simulink model "LIM_version_25052023"  (R2021a)
settings: Solver=VariableStepAuto  StartTime=0.0  StopTime=10.0  RelTol=1e-3
values from neighbouring files (symbols this model uses):
  ki_force = 1    [LIMvariables.m]
  ki_iedx = 80000    [LIMvariables.m]
  ki_ieqx = 80000    [LIMvariables.m]
  ki_lambda = 1000000    [LIMvariables.m]
  ki_speed = 10    [LIMvariables.m]
  kp_force = 0.15    [LIMvariables.m]
  kp_iedx = 25    [LIMvariables.m]
  kp_ieqx = 25    [LIMvariables.m]
  kp_lambda = 200    [LIMvariables.m]
  kp_speed = 0.1    [LIMvariables.m]
  l = 0.308    [LIMvariables.m]
  Llx = 0.0225    [LIMvariables.m]
  Lly = 0.0065    [LIMvariables.m]
  Lm = 0.0416    [LIM_parameters.m]    (also in LIMvariables.m = 0.0376)
  P = 4400    [LIMvariables.m]
  Rx = 1.2    [LIMvariables.m]
  Ry = 2.7    [LIMvariables.m]
  tau = L/p    (= 0.25)    [LIM_parameters.m]    (also in LIMvariables.m = 0.066)
undefined symbols (not defined in the file or in its folder): M, omega_e
libraries: slpidlib x5, simulink x3, simulink_extras x1
settings Model: Creator=Asus  LastModifiedBy=Asus

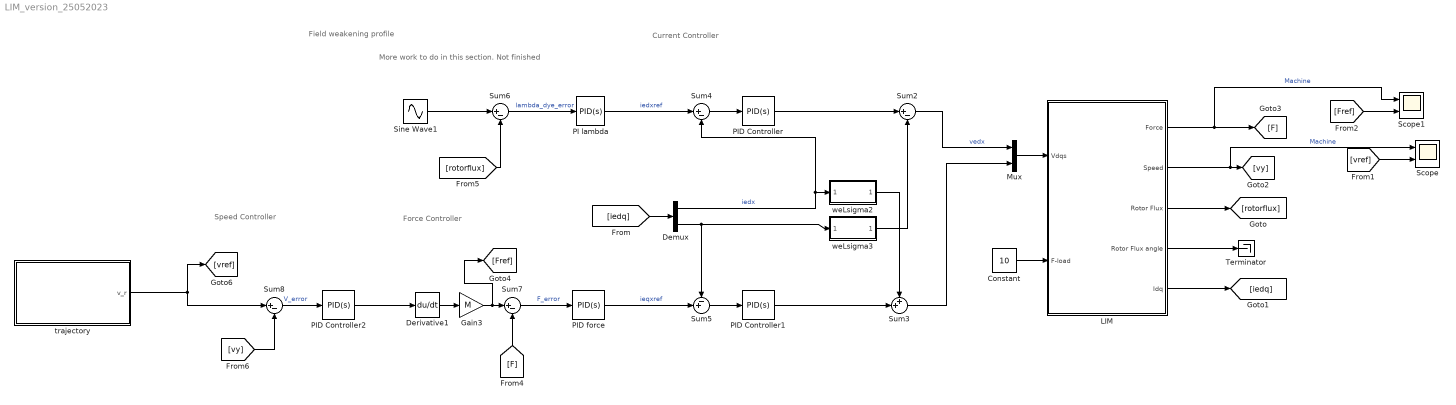
== system LIM_version_25052023 ==
  note: Current Controller
  note: Force Controller
  note: Field weakening profile
  note: Speed Controller
  note: More work to do in this section. Not finished
  Constant : Constant  Value=10
  Demux : Demux  Outputs=2
  Derivative1 : Derivative
  Gain3 : Gain  Gain=M
  LIM : Subsystem
  Mux : Mux  Inputs=2
  PI lambda : slpidlib/PID Controller  Controller=PID  Form=Parallel  TimeDomain=Continuous-time  UseExternalTs=off  SampleTime=-1  IntegratorMethod=Forward Euler  FilterMethod=Forward Euler  ControllerParametersSource=internal  P=kp_lambda  I=ki_lambda  D=0  UseFilter=on  N=100  TunerSelectOption=Transfer Function Based (PID Tuner App)  InitialConditionSource=internal  InitialConditionForIntegrator=0  InitialConditionForFilter=0  DifferentiatorICPrevScaledInput=0  ExternalReset=none  TrackingMode=off  Kt=1  LimitOutput=off  SatLimitsSource=internal  UpperSaturationLimit=inf  LowerSaturationLimit=-inf  LinearizeAsGain=on  AntiWindupMode=none  Kb=1  POutMin=[]  POutMax=[]  IOutMin=[]  IOutMax=[]  DOutMin=[]  DOutMax=[]  NOutMin=[]  NOutMax=[]  SumOutMin=[]  SumOutMax=[]  SaturationOutMin=[]  SaturationOutMax=[]  PParamMin=[]  PParamMax=[]  IParamMin=[]  IParamMax=[]  DParamMin=[]  DParamMax=[]  NParamMin=[]  NParamMax=[]  KbParamMin=[]  KbParamMax=[]  KtParamMin=[]  KtParamMax=[]  KbOutMin=[]  KbOutMax=[]  KtOutMin=[]  KtOutMax=[]  IntegratorOutMin=[]  IntegratorOutMax=[]  FilterOutMin=[]  FilterOutMax=[]  SumI1OutMin=[]  SumI1OutMax=[]  SumI2OutMin=[]  SumI2OutMax=[]  SumI3OutMin=[]  SumI3OutMax=[]  SumI4OutMin=[]  SumI4OutMax=[]  SumDOutMin=[]  SumDOutMax=[]  DifferentiatorOutMin=[]  DifferentiatorOutMax=[]  FilterDiffOutCoefMin=[]  FilterDiffOutCoefMax=[]  ReciprocalOutMin=[]  ReciprocalOutMax=[]  SumDenOutMin=[]  SumDenOutMax=[]  SumNumOutMin=[]  SumNumOutMax=[]  DivideOutMin=[]  DivideOutMax=[]  UdiffTsProdOutMin=[]  UdiffTsProdOutMax=[]  NTsProdOutMin=[]  NTsProdOutMax=[]  UintegralTsProdOutMin=[]  UintegralTsProdOutMax=[]  UngainTsProdOutMin=[]  UngainTsProdOutMax=[]  IntegratorContinuousStateAttributes=''  IntegratorStateMustResolveToSignalObject=off  IntegratorRTWStateStorageClass=Auto  FilterContinuousStateAttributes=''  FilterStateMustResolveToSignalObject=off  FilterRTWStateStorageClass=Auto  ParallelPVariant=InternalParameters  IdealPVariant=Disabled  IVariant=InternalParameters  DVariant=InternalParameters  IntegratorVariant=Continuous  SatVariant=Disabled  AWVariant=Passthrough  PCopyVariant=Disabled  TRVariant=Disabled  FdbkBlocksVariant=Forward  IdealPFdbkVariant=Disabled  SatFdbkVariant=Disabled  DerivativeFilterVariant=ContFilter  NVariant=InternalParameters  NCopyVariant=Disabled  FilterICVariant=InternalICsFilter  IntegratorICVariant=InternalICs  ExternalResetVariant=Disabled  TRSumVariant=Passthrough  SumFdbkVariant=Disabled  SumVariant=Sum_PID  TsampFilterVariant=InternalTs  TsampNgainVariant=Passthrough  TsampIntegralVariant=Passthrough  ExternalSaturationOutDataTypeStr=Inherit: Same as second input
  PID Controller : slpidlib/PID Controller  Controller=PID  Form=Parallel  TimeDomain=Continuous-time  UseExternalTs=off  SampleTime=-1  IntegratorMethod=Forward Euler  FilterMethod=Forward Euler  ControllerParametersSource=internal  P=kp_ieqx  I=ki_ieqx  D=0  UseFilter=on  N=100  TunerSelectOption=Transfer Function Based (PID Tuner App)  InitialConditionSource=internal  InitialConditionForIntegrator=0  InitialConditionForFilter=0  DifferentiatorICPrevScaledInput=0  ExternalReset=none  TrackingMode=off  Kt=1  LimitOutput=off  SatLimitsSource=internal  UpperSaturationLimit=inf  LowerSaturationLimit=-inf  LinearizeAsGain=on  AntiWindupMode=none  Kb=1  POutMin=[]  POutMax=[]  IOutMin=[]  IOutMax=[]  DOutMin=[]  DOutMax=[]  NOutMin=[]  NOutMax=[]  SumOutMin=[]  SumOutMax=[]  SaturationOutMin=[]  SaturationOutMax=[]  PParamMin=[]  PParamMax=[]  IParamMin=[]  IParamMax=[]  DParamMin=[]  DParamMax=[]  NParamMin=[]  NParamMax=[]  KbParamMin=[]  KbParamMax=[]  KtParamMin=[]  KtParamMax=[]  KbOutMin=[]  KbOutMax=[]  KtOutMin=[]  KtOutMax=[]  IntegratorOutMin=[]  IntegratorOutMax=[]  FilterOutMin=[]  FilterOutMax=[]  SumI1OutMin=[]  SumI1OutMax=[]  SumI2OutMin=[]  SumI2OutMax=[]  SumI3OutMin=[]  SumI3OutMax=[]  SumI4OutMin=[]  SumI4OutMax=[]  SumDOutMin=[]  SumDOutMax=[]  DifferentiatorOutMin=[]  DifferentiatorOutMax=[]  FilterDiffOutCoefMin=[]  FilterDiffOutCoefMax=[]  ReciprocalOutMin=[]  ReciprocalOutMax=[]  SumDenOutMin=[]  SumDenOutMax=[]  SumNumOutMin=[]  SumNumOutMax=[]  DivideOutMin=[]  DivideOutMax=[]  UdiffTsProdOutMin=[]  UdiffTsProdOutMax=[]  NTsProdOutMin=[]  NTsProdOutMax=[]  UintegralTsProdOutMin=[]  UintegralTsProdOutMax=[]  UngainTsProdOutMin=[]  UngainTsProdOutMax=[]  IntegratorContinuousStateAttributes=''  IntegratorStateMustResolveToSignalObject=off  IntegratorRTWStateStorageClass=Auto  FilterContinuousStateAttributes=''  FilterStateMustResolveToSignalObject=off  FilterRTWStateStorageClass=Auto  ParallelPVariant=InternalParameters  IdealPVariant=Disabled  IVariant=InternalParameters  DVariant=InternalParameters  IntegratorVariant=Continuous  SatVariant=Disabled  AWVariant=Passthrough  PCopyVariant=Disabled  TRVariant=Disabled  FdbkBlocksVariant=Forward  IdealPFdbkVariant=Disabled  SatFdbkVariant=Disabled  DerivativeFilterVariant=ContFilter  NVariant=InternalParameters  NCopyVariant=Disabled  FilterICVariant=InternalICsFilter  IntegratorICVariant=InternalICs  ExternalResetVariant=Disabled  TRSumVariant=Passthrough  SumFdbkVariant=Disabled  SumVariant=Sum_PID  TsampFilterVariant=InternalTs  TsampNgainVariant=Passthrough  TsampIntegralVariant=Passthrough  ExternalSaturationOutDataTypeStr=Inherit: Same as second input
  PID Controller1 : slpidlib/PID Controller  Controller=PID  Form=Parallel  TimeDomain=Continuous-time  UseExternalTs=off  SampleTime=-1  IntegratorMethod=Forward Euler  FilterMethod=Forward Euler  ControllerParametersSource=internal  P=kp_iedx  I=ki_iedx  D=0  UseFilter=on  N=100  TunerSelectOption=Transfer Function Based (PID Tuner App)  InitialConditionSource=internal  InitialConditionForIntegrator=0  InitialConditionForFilter=0  DifferentiatorICPrevScaledInput=0  ExternalReset=none  TrackingMode=off  Kt=1  LimitOutput=off  SatLimitsSource=internal  UpperSaturationLimit=inf  LowerSaturationLimit=-inf  LinearizeAsGain=on  AntiWindupMode=none  Kb=1  POutMin=[]  POutMax=[]  IOutMin=[]  IOutMax=[]  DOutMin=[]  DOutMax=[]  NOutMin=[]  NOutMax=[]  SumOutMin=[]  SumOutMax=[]  SaturationOutMin=[]  SaturationOutMax=[]  PParamMin=[]  PParamMax=[]  IParamMin=[]  IParamMax=[]  DParamMin=[]  DParamMax=[]  NParamMin=[]  NParamMax=[]  KbParamMin=[]  KbParamMax=[]  KtParamMin=[]  KtParamMax=[]  KbOutMin=[]  KbOutMax=[]  KtOutMin=[]  KtOutMax=[]  IntegratorOutMin=[]  IntegratorOutMax=[]  FilterOutMin=[]  FilterOutMax=[]  SumI1OutMin=[]  SumI1OutMax=[]  SumI2OutMin=[]  SumI2OutMax=[]  SumI3OutMin=[]  SumI3OutMax=[]  SumI4OutMin=[]  SumI4OutMax=[]  SumDOutMin=[]  SumDOutMax=[]  DifferentiatorOutMin=[]  DifferentiatorOutMax=[]  FilterDiffOutCoefMin=[]  FilterDiffOutCoefMax=[]  ReciprocalOutMin=[]  ReciprocalOutMax=[]  SumDenOutMin=[]  SumDenOutMax=[]  SumNumOutMin=[]  SumNumOutMax=[]  DivideOutMin=[]  DivideOutMax=[]  UdiffTsProdOutMin=[]  UdiffTsProdOutMax=[]  NTsProdOutMin=[]  NTsProdOutMax=[]  UintegralTsProdOutMin=[]  UintegralTsProdOutMax=[]  UngainTsProdOutMin=[]  UngainTsProdOutMax=[]  IntegratorContinuousStateAttributes=''  IntegratorStateMustResolveToSignalObject=off  IntegratorRTWStateStorageClass=Auto  FilterContinuousStateAttributes=''  FilterStateMustResolveToSignalObject=off  FilterRTWStateStorageClass=Auto  ParallelPVariant=InternalParameters  IdealPVariant=Disabled  IVariant=InternalParameters  DVariant=InternalParameters  IntegratorVariant=Continuous  SatVariant=Disabled  AWVariant=Passthrough  PCopyVariant=Disabled  TRVariant=Disabled  FdbkBlocksVariant=Forward  IdealPFdbkVariant=Disabled  SatFdbkVariant=Disabled  DerivativeFilterVariant=ContFilter  NVariant=InternalParameters  NCopyVariant=Disabled  FilterICVariant=InternalICsFilter  IntegratorICVariant=InternalICs  ExternalResetVariant=Disabled  TRSumVariant=Passthrough  SumFdbkVariant=Disabled  SumVariant=Sum_PID  TsampFilterVariant=InternalTs  TsampNgainVariant=Passthrough  TsampIntegralVariant=Passthrough  ExternalSaturationOutDataTypeStr=Inherit: Same as second input
  PID Controller2 : slpidlib/PID Controller  Controller=PID  Form=Parallel  TimeDomain=Continuous-time  UseExternalTs=off  SampleTime=-1  IntegratorMethod=Forward Euler  FilterMethod=Forward Euler  ControllerParametersSource=internal  P=kp_speed  I=ki_speed  D=0  UseFilter=on  N=100  TunerSelectOption=Transfer Function Based (PID Tuner App)  InitialConditionSource=internal  InitialConditionForIntegrator=0  InitialConditionForFilter=0  DifferentiatorICPrevScaledInput=0  ExternalReset=none  TrackingMode=off  Kt=1  LimitOutput=off  SatLimitsSource=internal  UpperSaturationLimit=inf  LowerSaturationLimit=-inf  LinearizeAsGain=on  AntiWindupMode=none  Kb=1  POutMin=[]  POutMax=[]  IOutMin=[]  IOutMax=[]  DOutMin=[]  DOutMax=[]  NOutMin=[]  NOutMax=[]  SumOutMin=[]  SumOutMax=[]  SaturationOutMin=[]  SaturationOutMax=[]  PParamMin=[]  PParamMax=[]  IParamMin=[]  IParamMax=[]  DParamMin=[]  DParamMax=[]  NParamMin=[]  NParamMax=[]  KbParamMin=[]  KbParamMax=[]  KtParamMin=[]  KtParamMax=[]  KbOutMin=[]  KbOutMax=[]  KtOutMin=[]  KtOutMax=[]  IntegratorOutMin=[]  IntegratorOutMax=[]  FilterOutMin=[]  FilterOutMax=[]  SumI1OutMin=[]  SumI1OutMax=[]  SumI2OutMin=[]  SumI2OutMax=[]  SumI3OutMin=[]  SumI3OutMax=[]  SumI4OutMin=[]  SumI4OutMax=[]  SumDOutMin=[]  SumDOutMax=[]  DifferentiatorOutMin=[]  DifferentiatorOutMax=[]  FilterDiffOutCoefMin=[]  FilterDiffOutCoefMax=[]  ReciprocalOutMin=[]  ReciprocalOutMax=[]  SumDenOutMin=[]  SumDenOutMax=[]  SumNumOutMin=[]  SumNumOutMax=[]  DivideOutMin=[]  DivideOutMax=[]  UdiffTsProdOutMin=[]  UdiffTsProdOutMax=[]  NTsProdOutMin=[]  NTsProdOutMax=[]  UintegralTsProdOutMin=[]  UintegralTsProdOutMax=[]  UngainTsProdOutMin=[]  UngainTsProdOutMax=[]  IntegratorContinuousStateAttributes=''  IntegratorStateMustResolveToSignalObject=off  IntegratorRTWStateStorageClass=Auto  FilterContinuousStateAttributes=''  FilterStateMustResolveToSignalObject=off  FilterRTWStateStorageClass=Auto  ParallelPVariant=InternalParameters  IdealPVariant=Disabled  IVariant=InternalParameters  DVariant=InternalParameters  IntegratorVariant=Continuous  SatVariant=Disabled  AWVariant=Passthrough  PCopyVariant=Disabled  TRVariant=Disabled  FdbkBlocksVariant=Forward  IdealPFdbkVariant=Disabled  SatFdbkVariant=Disabled  DerivativeFilterVariant=ContFilter  NVariant=InternalParameters  NCopyVariant=Disabled  FilterICVariant=InternalICsFilter  IntegratorICVariant=InternalICs  ExternalResetVariant=Disabled  TRSumVariant=Passthrough  SumFdbkVariant=Disabled  SumVariant=Sum_PID  TsampFilterVariant=InternalTs  TsampNgainVariant=Passthrough  TsampIntegralVariant=Passthrough  ExternalSaturationOutDataTypeStr=Inherit: Same as second input
  PID force : slpidlib/PID Controller  Controller=PID  Form=Parallel  TimeDomain=Continuous-time  UseExternalTs=off  SampleTime=-1  IntegratorMethod=Forward Euler  FilterMethod=Forward Euler  ControllerParametersSource=internal  P=kp_force  I=ki_force  D=0  UseFilter=on  N=100  TunerSelectOption=Transfer Function Based (PID Tuner App)  InitialConditionSource=internal  InitialConditionForIntegrator=0  InitialConditionForFilter=0  DifferentiatorICPrevScaledInput=0  ExternalReset=none  TrackingMode=off  Kt=1  LimitOutput=off  SatLimitsSource=internal  UpperSaturationLimit=inf  LowerSaturationLimit=-inf  LinearizeAsGain=on  AntiWindupMode=none  Kb=1  POutMin=[]  POutMax=[]  IOutMin=[]  IOutMax=[]  DOutMin=[]  DOutMax=[]  NOutMin=[]  NOutMax=[]  SumOutMin=[]  SumOutMax=[]  SaturationOutMin=[]  SaturationOutMax=[]  PParamMin=[]  PParamMax=[]  IParamMin=[]  IParamMax=[]  DParamMin=[]  DParamMax=[]  NParamMin=[]  NParamMax=[]  KbParamMin=[]  KbParamMax=[]  KtParamMin=[]  KtParamMax=[]  KbOutMin=[]  KbOutMax=[]  KtOutMin=[]  KtOutMax=[]  IntegratorOutMin=[]  IntegratorOutMax=[]  FilterOutMin=[]  FilterOutMax=[]  SumI1OutMin=[]  SumI1OutMax=[]  SumI2OutMin=[]  SumI2OutMax=[]  SumI3OutMin=[]  SumI3OutMax=[]  SumI4OutMin=[]  SumI4OutMax=[]  SumDOutMin=[]  SumDOutMax=[]  DifferentiatorOutMin=[]  DifferentiatorOutMax=[]  FilterDiffOutCoefMin=[]  FilterDiffOutCoefMax=[]  ReciprocalOutMin=[]  ReciprocalOutMax=[]  SumDenOutMin=[]  SumDenOutMax=[]  SumNumOutMin=[]  SumNumOutMax=[]  DivideOutMin=[]  DivideOutMax=[]  UdiffTsProdOutMin=[]  UdiffTsProdOutMax=[]  NTsProdOutMin=[]  NTsProdOutMax=[]  UintegralTsProdOutMin=[]  UintegralTsProdOutMax=[]  UngainTsProdOutMin=[]  UngainTsProdOutMax=[]  IntegratorContinuousStateAttributes=''  IntegratorStateMustResolveToSignalObject=off  IntegratorRTWStateStorageClass=Auto  FilterContinuousStateAttributes=''  FilterStateMustResolveToSignalObject=off  FilterRTWStateStorageClass=Auto  ParallelPVariant=InternalParameters  IdealPVariant=Disabled  IVariant=InternalParameters  DVariant=InternalParameters  IntegratorVariant=Continuous  SatVariant=Disabled  AWVariant=Passthrough  PCopyVariant=Disabled  TRVariant=Disabled  FdbkBlocksVariant=Forward  IdealPFdbkVariant=Disabled  SatFdbkVariant=Disabled  DerivativeFilterVariant=ContFilter  NVariant=InternalParameters  NCopyVariant=Disabled  FilterICVariant=InternalICsFilter  IntegratorICVariant=InternalICs  ExternalResetVariant=Disabled  TRSumVariant=Passthrough  SumFdbkVariant=Disabled  SumVariant=Sum_PID  TsampFilterVariant=InternalTs  TsampNgainVariant=Passthrough  TsampIntegralVariant=Passthrough  ExternalSaturationOutDataTypeStr=Inherit: Same as second input
  Scope : Scope  NumInputPorts=2
  Scope1 : Scope  NumInputPorts=2
  Sine Wave1 : Sin  Amplitude=10  SampleTime=0
  Sum{2,4,6..8} (5 alike) : Sum  Inputs=|+-
  Sum3 : Sum  Inputs=++|
  Sum5 : Sum  Inputs=-+|
  Terminator : Terminator
  trajectory : Subsystem
  weLsigma2 : Subsystem
  weLsigma3 : Subsystem
  wires:
  trajectory/1(v_r) -> Sum8/1, [vref]
  PID force/1 -> Sum5/2  "ieqxref"
  weLsigma3/1(Out1) -> Sum2/2
  Sine Wave1/1 -> Sum6/1
  weLsigma2/1(Out1) -> Sum3/1
  Sum5/1 -> PID Controller1/1
  [rotorflux] -> Sum6/2
  [vy] -> Sum8/2
  Sum7/1 -> PID force/1  "F_error"
  Sum2/1 -> Mux/1  "vedx"
  PID Controller/1 -> Sum2/1
  Derivative1/1 -> Gain3/1
  Gain3/1 -> [Fref], Sum7/1
  [F] -> Sum7/2
  PID Controller2/1 -> Derivative1/1
  PI lambda/1 -> Sum4/1  "iedxref"
  Sum3/1 -> Mux/2
  PID Controller1/1 -> Sum3/2
  Sum4/1 -> PID Controller/1
  Demux/1 -> Sum4/2, weLsigma2/1(Input)  "iedx"
  Sum8/1 -> PID Controller2/1  "V_error"
  Sum6/1 -> PI lambda/1  "lambda_dye_error"
  LIM/3(" Rotor Flux") -> [rotorflux]
  LIM/5(" Idq") -> [iedq]
  [iedq] -> Demux/1
  Demux/2 -> Sum5/1, weLsigma3/1(Input)
  Mux/1 -> LIM/1(Vdqs)
  Constant/1 -> LIM/2(F-load)
  LIM/2(" Speed") -> Scope/1, [vy]  "Machine"
  LIM/4(" Rotor Flux angle") -> Terminator/1
  [vref] -> Scope/2
  LIM/1("Force ") -> Scope1/1, [F]  "Machine"
  [Fref] -> Scope1/2

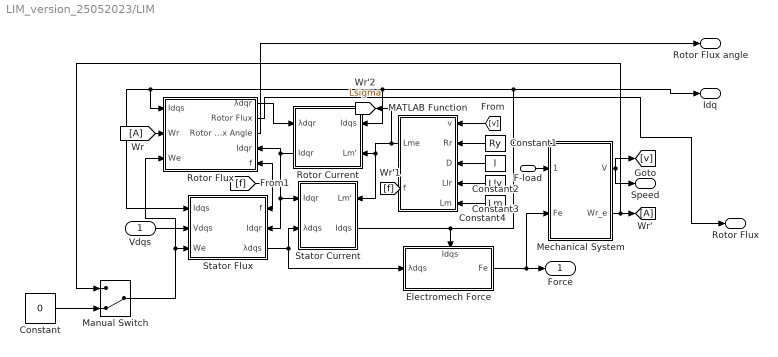
== system LIM_version_25052023/LIM ==
  Vdqs : Inport
  F-load : Inport  Port=2
  Constant : Constant  Value=0
  Constant1 : Constant  Value=Ry
  Constant2 : Constant  Value=l
  Constant3 : Constant  Value=Lly
  Constant4 : Constant  Value=Lm
  Electromech Force : Subsystem
      settings: PortSchema="{\"entries\":[{\"content\":{\"sides\":[{\"content\":{\"connectorIds\":[\"In1\"]},\"type\":\"ConnectorPlacement.EquallySpacedRectSide\",\"uuid\":\"a4b29cca-9cb0-4324-9244-2049ffc93668\"},{\"content\":{\"connectorIds\":[\"Out1\"],\"side\":\"RIGHT\"},\"type\":\"ConnectorPlacement.EquallySpacedRectSide\",\"uuid\":\"b20ff3ac-d40e-4f59-bb91-f6f2c0c6ca63\"},{\"content\":{\"connectorIds\":[\"In2\"],\"side\":\"TOP\"},\"type\":\"ConnectorPlacement.EquallySpacedRectSide\",\"uuid\":\"55342d43-b8f9-4aa9-846c-26670e92f4ca\"},{\"content\":{\"connectorIds\":[],\"side\":\"HIDDEN\"},\"type\":\"ConnectorPlacement.EquallySpacedRectSide\",\"uuid\":\"5fed22a0-a45a-430c-a997-0be85a9315bb\"}]},\"type\":\"ConnectorPlacement.EquallySpacedConnector\",\"uuid\":\"78d5652d-2b6b-4c50-974b-d09ad892483f\"}],\"packageUris\":[\"http://schema.mathworks.com/mf0/Connector/R2020b\"],\"version\":\"1.0\"}"
  MATLAB Function : MATLAB Function  TreatAsAtomicUnit=on
  Manual Switch : ManualSwitch  CurrentSetting=0
  Mechanical System : Subsystem
  Rotor Current : Subsystem
      settings: PortSchema="{\"entries\":[{\"content\":{\"sides\":[{\"content\":{\"connectorIds\":[\"In1\",\"Out1\"]},\"type\":\"ConnectorPlacement.EquallySpacedRectSide\",\"uuid\":\"b9a9f404-9b3b-4182-a50e-1bf7cef191e8\"},{\"content\":{\"connectorIds\":[\"In2\",\"In3\"],\"side\":\"RIGHT\"},\"type\":\"ConnectorPlacement.EquallySpacedRectSide\",\"uuid\":\"68159d79-7975-4fd0-98a3-7e35432781a2\"},{\"content\":{\"connectorIds\":[],\"side\":\"TOP\"},\"type\":\"ConnectorPlacement.EquallySpacedRectSide\",\"uuid\":\"0c4dbb5d-b4d4-4876-b829-49090bd6eeb8\"},{\"content\":{\"connectorIds\":[],\"side\":\"BOTTOM\"},\"type\":\"ConnectorPlacement.EquallySpacedRectSide\",\"uuid\":\"e42509db-2e5f-42f8-9a91-9046ba95e836\"},{\"content\":{\"connectorIds\":[],\"side\":\"HIDDEN\"},\"type\":\"ConnectorPlacement.EquallySpacedRectSide\",\"uuid\":\"f2a65973-682a-4dd6-b429-3fa72198cae4\"}]},\"type\":\"ConnectorPlacement.EquallySpacedConnector\",\"uuid\":\"744eb17f-cf6a-4151-90db-78263b57d619\"}],\"packageUris\":[\"http://schema.mathworks.com/mf0/Connector/R2020b\"],\"version\":\"1.0\"}"
  Rotor Flux : Subsystem
      settings: PortSchema="{\"entries\":[{\"content\":{\"sides\":[{\"content\":{\"connectorIds\":[\"In1\",\"In2\",\"In3\"]},\"type\":\"ConnectorPlacement.EquallySpacedRectSide\",\"uuid\":\"b9a9f404-9b3b-4182-a50e-1bf7cef191e8\"},{\"content\":{\"connectorIds\":[\"Out1\",\"Out2\",\"Out3\",\"In4\",\"In5\"],\"side\":\"RIGHT\"},\"type\":\"ConnectorPlacement.EquallySpacedRectSide\",\"uuid\":\"68159d79-7975-4fd0-98a3-7e35432781a2\"},{\"content\":{\"connectorIds\":[],\"side\":\"TOP\"},\"type\":\"ConnectorPlacement.EquallySpacedRectSide\",\"uuid\":\"0c4dbb5d-b4d4-4876-b829-49090bd6eeb8\"},{\"content\":{\"connectorIds\":[],\"side\":\"HIDDEN\"},\"type\":\"ConnectorPlacement.EquallySpacedRectSide\",\"uuid\":\"f2a65973-682a-4dd6-b429-3fa72198cae4\"}]},\"type\":\"ConnectorPlacement.EquallySpacedConnector\",\"uuid\":\"744eb17f-cf6a-4151-90db-78263b57d619\"}],\"packageUris\":[\"http://schema.mathworks.com/mf0/Connector/R2020b\"],\"version\":\"1.0\"}"
  Stator Current : Subsystem
      settings: PortSchema="{\"entries\":[{\"content\":{\"sides\":[{\"content\":{\"connectorIds\":[\"In1\",\"In2\"]},\"type\":\"ConnectorPlacement.EquallySpacedRectSide\",\"uuid\":\"c6a8d684-b7d2-4173-9e8a-0a77b360fa3b\"},{\"content\":{\"connectorIds\":[\"In3\",\"Out1\"],\"side\":\"RIGHT\"},\"type\":\"ConnectorPlacement.EquallySpacedRectSide\",\"uuid\":\"6b547613-238c-47a7-9a25-113e0bcf67e8\"},{\"content\":{\"connectorIds\":[],\"side\":\"TOP\"},\"type\":\"ConnectorPlacement.EquallySpacedRectSide\",\"uuid\":\"9eb731ca-d22d-4bff-90d4-9f452150afc4\"},{\"content\":{\"connectorIds\":[],\"side\":\"HIDDEN\"},\"type\":\"ConnectorPlacement.EquallySpacedRectSide\",\"uuid\":\"3386087c-4273-46bf-b0bc-9959c9fde15b\"}]},\"type\":\"ConnectorPlacement.EquallySpacedConnector\",\"uuid\":\"3fded039-aa6e-4722-8a98-01f4cd5eabc0\"}],\"packageUris\":[\"http://schema.mathworks.com/mf0/Connector/R2020b\"],\"version\":\"1.0\"}"
  Stator Flux : Subsystem
      settings: PortSchema="{\"entries\":[{\"content\":{\"sides\":[{\"content\":{\"connectorIds\":[\"In1\",\"In2\",\"In3\"]},\"type\":\"ConnectorPlacement.EquallySpacedRectSide\",\"uuid\":\"a4b29cca-9cb0-4324-9244-2049ffc93668\"},{\"content\":{\"connectorIds\":[\"In4\",\"In5\",\"Out1\"],\"side\":\"RIGHT\"},\"type\":\"ConnectorPlacement.EquallySpacedRectSide\",\"uuid\":\"b20ff3ac-d40e-4f59-bb91-f6f2c0c6ca63\"},{\"content\":{\"connectorIds\":[],\"side\":\"TOP\"},\"type\":\"ConnectorPlacement.EquallySpacedRectSide\",\"uuid\":\"55342d43-b8f9-4aa9-846c-26670e92f4ca\"},{\"content\":{\"connectorIds\":[],\"side\":\"HIDDEN\"},\"type\":\"ConnectorPlacement.EquallySpacedRectSide\",\"uuid\":\"5fed22a0-a45a-430c-a997-0be85a9315bb\"}]},\"type\":\"ConnectorPlacement.EquallySpacedConnector\",\"uuid\":\"78d5652d-2b6b-4c50-974b-d09ad892483f\"}],\"packageUris\":[\"http://schema.mathworks.com/mf0/Connector/R2020b\"],\"version\":\"1.0\"}"
  "Force " : Outport
  " Speed" : Outport  Port=2
  " Rotor Flux" : Outport  Port=3
  " Rotor Flux angle" : Outport  Port=4
  " Idq" : Outport  Port=5
  tag scope: Lsigma=global
  wires:
  Electromech Force/1(Fe) -> Mechanical System/2(Fe), "Force "/1
  F-load/1 -> Mechanical System/1(F-load)
  Mechanical System/1(V) -> " Speed"/1, [v]
  Stator Flux/1(λdqs) -> Stator Current/2(λdqs), Electromech Force/1(λdqs)
  Stator Current/1(Idqs) -> Electromech Force/2(Idqs), " Idq"/1, Rotor Flux/1(Idqs), Stator Flux/1(Idqs), Rotor Current/2(Idqs)
  Rotor Flux/1(λdqr) -> Rotor Current/1(λdqr)
  Rotor Current/1(Idqr) -> Rotor Flux/4(Idqr), Stator Flux/5(Idqr), Stator Current/1(Idqr)
  [A] -> Rotor Flux/2(Wr)
  MATLAB Function/1(Lme) -> Stator Current/3(Lm'), Rotor Current/3(Lm'), [Lsigma]
  [v] -> MATLAB Function/1(v)
  Constant1/1 -> MATLAB Function/2(Rr)
  Constant2/1 -> MATLAB Function/3(D)
  Constant3/1 -> MATLAB Function/4(Llr)
  Constant4/1 -> MATLAB Function/5(Lm)
  MATLAB Function/2(f) -> [f]
  [f] -> Rotor Flux/5(f), Stator Flux/4(f)
  Mechanical System/2(Wr_e) -> Manual Switch/1, [A]
  Manual Switch/1 -> Rotor Flux/3(We), Stator Flux/3(We)
  Constant/1 -> Manual Switch/2
  Rotor Flux/2(Rotor Flux) -> " Rotor Flux"/1
  Rotor Flux/3(Rotor Flux Angle) -> " Rotor Flux angle"/1
  Vdqs/1 -> Stator Flux/2(Vdqs)

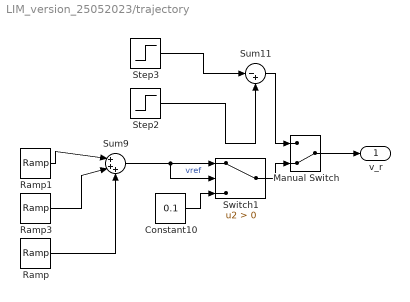
== system LIM_version_25052023/trajectory ==
  Constant10 : Constant  Value=0.1
  Manual Switch : ManualSwitch  CurrentSetting=0
  Ramp : simulink/Sources/Ramp  slope=-6.5  start=5.28  InitialOutput=0
  Ramp1 : simulink/Sources/Ramp  slope=4.12  start=0  InitialOutput=0.1
  Ramp3 : simulink/Sources/Ramp  slope=-4.4  start=5.28  InitialOutput=0.1
  Step2 : Step  Time=0  Before=0.1  After=20  SampleTime=0
  Step3 : Step  Time=4  Before=20  After=0.1  SampleTime=0
  Sum11 : Sum  Inputs=|-+
  Sum9 : Sum  Inputs=|+++
  Switch1 : Switch  Criteria=u2 > Threshold
  v_r : Outport
  wires:
  Switch1/1 -> Manual Switch/2
  Sum11/1 -> Manual Switch/1
  Constant10/1 -> Switch1/3
  Ramp3/1 -> Sum9/2
  Step2/1 -> Sum11/2
  Ramp/1 -> Sum9/3
  Step3/1 -> Sum11/1
  Ramp1/1 -> Sum9/1
  Sum9/1 -> Switch1/1, Switch1/2  "vref"
  Manual Switch/1 -> v_r/1

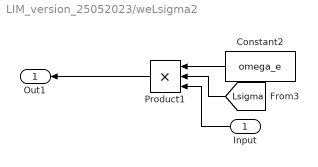
== system LIM_version_25052023/weLsigma2 ==
  Input : Inport
  Constant2 : Constant  Value=omega_e
  Product1 : Product  Inputs=3
  Out1 : Outport
  wires:
  Product1/1 -> Out1/1
  Constant2/1 -> Product1/1
  [Lsigma] -> Product1/2
  Input/1 -> Product1/3

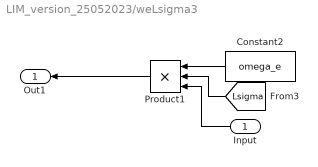
== system LIM_version_25052023/weLsigma3 ==
  Input : Inport
  Constant2 : Constant  Value=omega_e
  Product1 : Product  Inputs=3
  Out1 : Outport
  wires:
  Product1/1 -> Out1/1
  Constant2/1 -> Product1/1
  [Lsigma] -> Product1/2
  Input/1 -> Product1/3

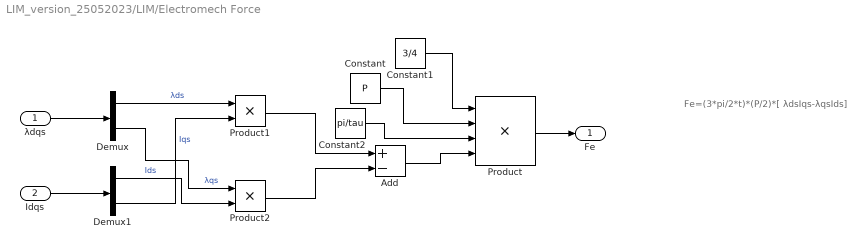
== system LIM_version_25052023/LIM/Electromech Force ==
  note: Fe=(3*pi/2*t)*(P/2)*[ λdsIqs-λqsIds]
  λdqs : Inport
  Idqs : Inport  Port=2
  Add : Sum  Inputs=+-
  Constant : Constant  Value=P
  Constant1 : Constant  Value=3/4
  Constant2 : Constant  Value=pi/tau
  Demux : Demux  Outputs=2
  Demux1 : Demux  Outputs=2
  Product : Product  Inputs=4
  Product1 : Product
  Product2 : Product
  Fe : Outport
  wires:
  Product/1 -> Fe/1
  Constant1/1 -> Product/1
  Constant/1 -> Product/2
  λdqs/1 -> Demux/1
  Idqs/1 -> Demux1/1
  Add/1 -> Product/4
  Demux/1 -> Product1/1  "λds"
  Demux1/2 -> Product1/2  "Iqs"
  Demux/2 -> Product2/1  "λqs"
  Demux1/1 -> Product2/2  "Ids"
  Product1/1 -> Add/1
  Product2/1 -> Add/2
  Constant2/1 -> Product/3

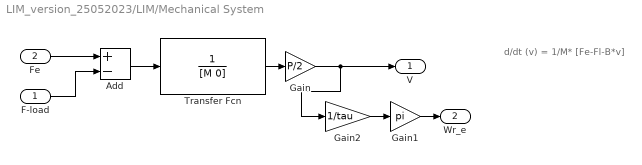
== system LIM_version_25052023/LIM/Mechanical System ==
  note: d/dt (v) = 1/M* [Fe-Fl-B*v]
  F-load : Inport
  Fe : Inport  Port=2
  Add : Sum  Inputs=+-
  Gain : Gain  Gain=P/2
  Gain1 : Gain  Gain=pi
  Gain2 : Gain  Gain=1/tau
  Transfer Fcn : TransferFcn  Denominator=[M 0]
  V : Outport
  Wr_e : Outport  Port=2
  wires:
  Fe/1 -> Add/1
  F-load/1 -> Add/2
  Add/1 -> Transfer Fcn/1
  Gain2/1 -> Gain1/1
  Gain1/1 -> Wr_e/1
  Gain/1 -> Gain2/1, V/1
  Transfer Fcn/1 -> Gain/1

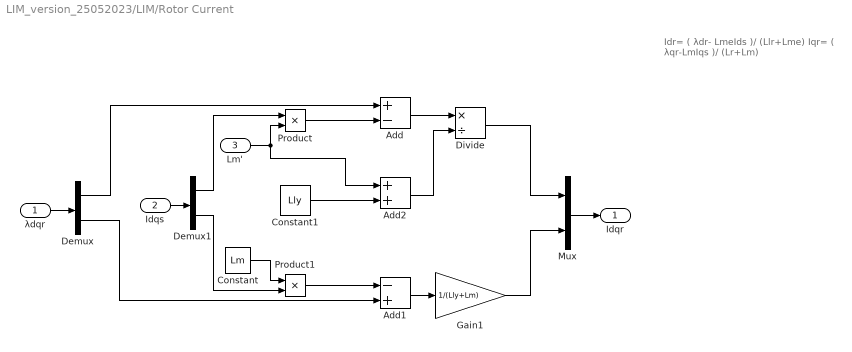
== system LIM_version_25052023/LIM/Rotor Current ==
  note: Idr= ( λdr- LmeIds )/ (Llr+Lme)
      |
      | Iqr= ( λqr-LmIqs )/ (Lr+Lm)
  λdqr : Inport
  Idqs : Inport  Port=2
  Lm' : Inport  Port=3
  Add : Sum  Inputs=+-
  Add1 : Sum  Inputs=-+
  Add2 : Sum
  Constant : Constant  Value=Lm  VectorParams1D=off
  Constant1 : Constant  Value=Lly
  Demux : Demux  Outputs=2
  Demux1 : Demux  Outputs=2
  Divide : Product  Inputs=*/
  Gain1 : Gain  Gain=1/(Lly+Lm)
  Mux : Mux  Inputs=2
  Product : Product
  Product1 : Product
  Idqr : Outport
  wires:
  Mux/1 -> Idqr/1
  λdqr/1 -> Demux/1
  Idqs/1 -> Demux1/1
  Demux1/1 -> Product/1
  Demux1/2 -> Product1/2
  Demux/1 -> Add/1
  Demux/2 -> Add1/2
  Product/1 -> Add/2
  Product1/1 -> Add1/1
  Add/1 -> Divide/1
  Add1/1 -> Gain1/1
  Gain1/1 -> Mux/2
  Divide/1 -> Mux/1
  Constant/1 -> Product1/1
  Constant1/1 -> Add2/2
  Lm'/1 -> Add2/1, Product/2
  Add2/1 -> Divide/2

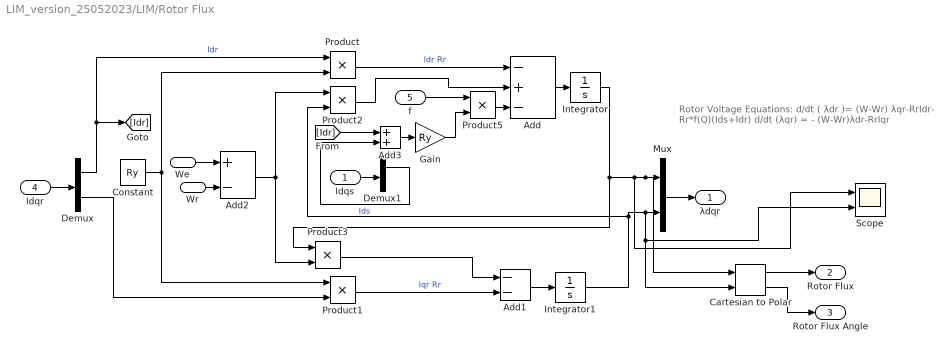
== system LIM_version_25052023/LIM/Rotor Flux ==
  note: Rotor Voltage Equations:
      | d/dt ( λdr )= (W-Wr) λqr-RrIdr- Rr*f(Q)(Ids+Idr)
      | d/dt (λqr) = - (W-Wr)λdr-RrIqr
  Idqs : Inport
  Wr : Inport  Port=2
  We : Inport  Port=3
  Idqr : Inport  Port=4
  f : Inport  Port=5
  Add : Sum  Inputs=-+-
  Add1 : Sum  Inputs=--
  Add2 : Sum  Inputs=+-
  Add3 : Sum
  Cartesian to Polar : simulink_extras/Transformations/Cartesian to Polar
  Constant : Constant  Value=Ry
  Demux : Demux  Outputs=2
  Demux1 : Demux  Outputs=2
  Gain : Gain  Gain=Ry
  Integrator : Integrator
  Integrator1 : Integrator
  Mux : Mux  Inputs=2
  Product{,1..3,5} (5 alike) : Product
  Scope : Scope  NumInputPorts=2
  λdqr : Outport
  Rotor Flux : Outport  Port=2
  Rotor Flux Angle : Outport  Port=3
  wires:
  Mux/1 -> λdqr/1
  Idqr/1 -> Demux/1
  Demux/1 -> [Idr], Product/1  "Idr"
  Demux/2 -> Product1/2
  Constant/1 -> Product1/1, Product/2
  Product/1 -> Add/1  "Idr Rr"
  Product1/1 -> Add1/2  "Iqr Rr"
  Add/1 -> Integrator/1
  Add1/1 -> Integrator1/1
  We/1 -> Add2/1
  Wr/1 -> Add2/2
  Add2/1 -> Product3/2, Product2/1
  Product2/1 -> Add/2
  Product3/1 -> Add1/1
  Demux1/1 -> Add3/2  "Ids"
  Product5/1 -> Add/3
  Add3/1 -> Gain/1
  Gain/1 -> Product5/2
  f/1 -> Product5/1
  Idqs/1 -> Demux1/1
  [Idr] -> Add3/1
  Cartesian to Polar/1 -> Rotor Flux/1
  Cartesian to Polar/2 -> Rotor Flux Angle/1
  Integrator1/1 -> Scope/2, Cartesian to Polar/2, Mux/2, Product2/2
  Integrator/1 -> Product3/1, Scope/1, Cartesian to Polar/1, Mux/1

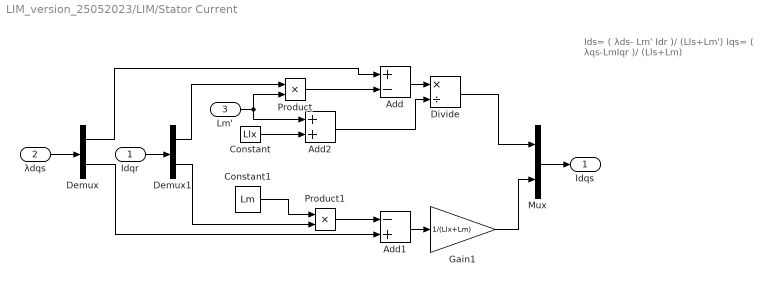
== system LIM_version_25052023/LIM/Stator Current ==
  note: Ids= ( λds- Lm' Idr )/ (Lls+Lm')
      |
      | Iqs= ( λqs-LmIqr )/ (Lls+Lm)
  Idqr : Inport
  λdqs : Inport  Port=2
  Lm' : Inport  Port=3
  Add : Sum  Inputs=+-
  Add1 : Sum  Inputs=-+
  Add2 : Sum
  Constant : Constant  Value=Llx
  Constant1 : Constant  Value=Lm  VectorParams1D=off
  Demux : Demux  Outputs=2
  Demux1 : Demux  Outputs=2
  Divide : Product  Inputs=*/
  Gain1 : Gain  Gain=1/(Llx+Lm)
  Mux : Mux  Inputs=2
  Product : Product
  Product1 : Product
  Idqs : Outport
  wires:
  Demux/2 -> Add1/2
  Demux1/1 -> Product/1
  Product/1 -> Add/2
  Product1/1 -> Add1/1
  λdqs/1 -> Demux/1
  Add1/1 -> Gain1/1
  Mux/1 -> Idqs/1
  Idqr/1 -> Demux1/1
  Demux/1 -> Add/1
  Demux1/2 -> Product1/2
  Add/1 -> Divide/1
  Divide/1 -> Mux/1
  Gain1/1 -> Mux/2
  Constant1/1 -> Product1/1
  Lm'/1 -> Add2/1, Product/2
  Constant/1 -> Add2/2
  Add2/1 -> Divide/2

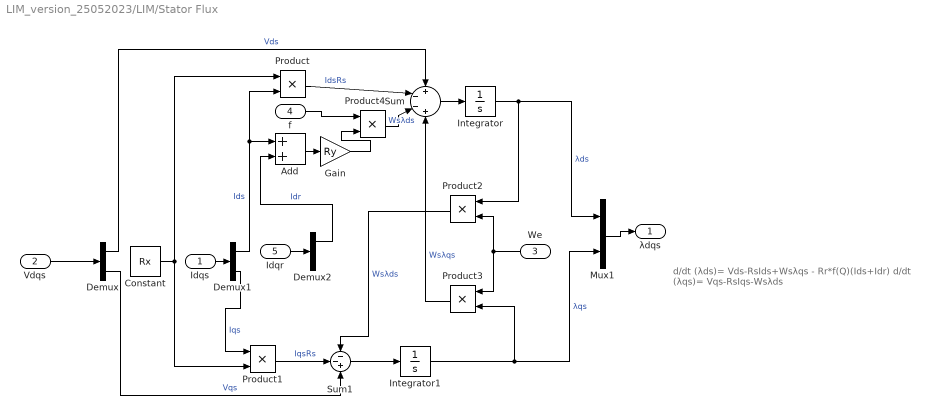
== system LIM_version_25052023/LIM/Stator Flux ==
  note: d/dt (λds)= Vds-RsIds+Wsλqs - Rr*f(Q)(Ids+Idr)
      |
      | d/dt (λqs)= Vqs-RsIqs-Wsλds
  Idqs : Inport
  Vdqs : Inport  Port=2
  We : Inport  Port=3
  f : Inport  Port=4
  Idqr : Inport  Port=5
  Add : Sum
  Constant : Constant  Value=Rx
  Demux : Demux  Outputs=2
  Demux1 : Demux  Outputs=2
  Demux2 : Demux  Outputs=2
  Gain : Gain  Gain=Ry
  Integrator : Integrator
  Integrator1 : Integrator
  Mux1 : Mux  Inputs=2
  Product{,1..4} (5 alike) : Product
  Sum : Sum  Inputs=+--+
  Sum1 : Sum  Inputs=--+
  λdqs : Outport
  wires:
  Integrator1/1 -> Product3/2, Mux1/2  "λqs"
  Integrator/1 -> Product2/1, Mux1/1  "λds"
  Vdqs/1 -> Demux/1
  Idqs/1 -> Demux1/1
  Demux/1 -> Sum/1  "Vds"
  Sum/1 -> Integrator/1
  Constant/1 -> Product1/2, Product/1
  Demux1/1 -> Product/2, Add/1  "Ids"
  Product/1 -> Sum/2  "IdsRs"
  Sum1/1 -> Integrator1/1
  Demux/2 -> Sum1/3  "Vqs"
  Demux1/2 -> Product1/1  "Iqs"
  Product1/1 -> Sum1/2  "IqsRs"
  We/1 -> Product3/1, Product2/2
  Product3/1 -> Sum/4  "Wsλqs"
  Product2/1 -> Sum1/1  "Wsλds"
  Mux1/1 -> λdqs/1
  Idqr/1 -> Demux2/1
  Demux2/1 -> Add/2  "Idr"
  Add/1 -> Gain/1
  Gain/1 -> Product4/2
  Product4/1 -> Sum/3  "Wsλds"
  f/1 -> Product4/1

== matlab function LIM_version_25052023/LIM/MATLAB Function ==
  data: v input; Lme output; Rr input; D input; Llr input; Lm input; f output
function [Lme,f]= fcn(v, Rr,D,Llr,Lm)
Q=abs((D*Rr)/(Llr*v));
f=(1-(exp(-Q)))/Q;
Lme = Lm*(1-f)
